simulink model "lab_1_2"  (R2019a)
settings: Solver=VariableStepAuto  StartTime=0.0  StopTime=10.0  RelTol=1e-3
settings Model: Creator=ADMIN  LastModifiedBy=ADMIN

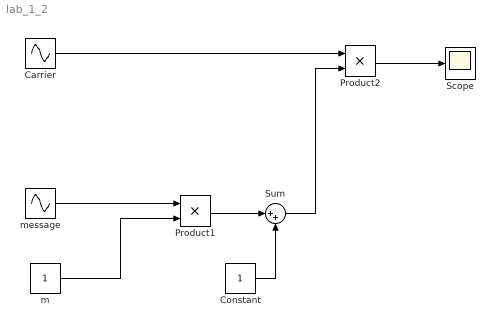
== system lab_1_2 ==
  Carrier : Sin  Frequency=2*pi*25  SampleTime=1/5000
  Constant : Constant
  Product1 : Product
  Product2 : Product
  Scope : Scope
  Sum : Sum  Inputs=|++
  "m " : Constant
  "message " : Sin  Bias=2*pi  SampleTime=1/5000
  wires:
  "message "/1 -> Product1/1
  "m "/1 -> Product1/2
  Carrier/1 -> Product2/1
  Product1/1 -> Sum/1
  Sum/1 -> Product2/2
  Constant/1 -> Sum/2
  Product2/1 -> Scope/1
